simulink model "cartpole_with_obsever"  (R2023a)
settings: Solver=ode45  StartTime=0.0  StopTime=10  RelTol=1e-3
settings Model: Creator=HW  LastModifiedBy=HW

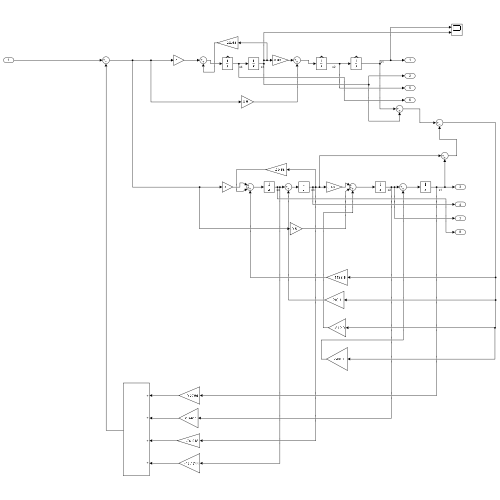
[thumbnail: Simulink's stored preview of the top-level diagram]
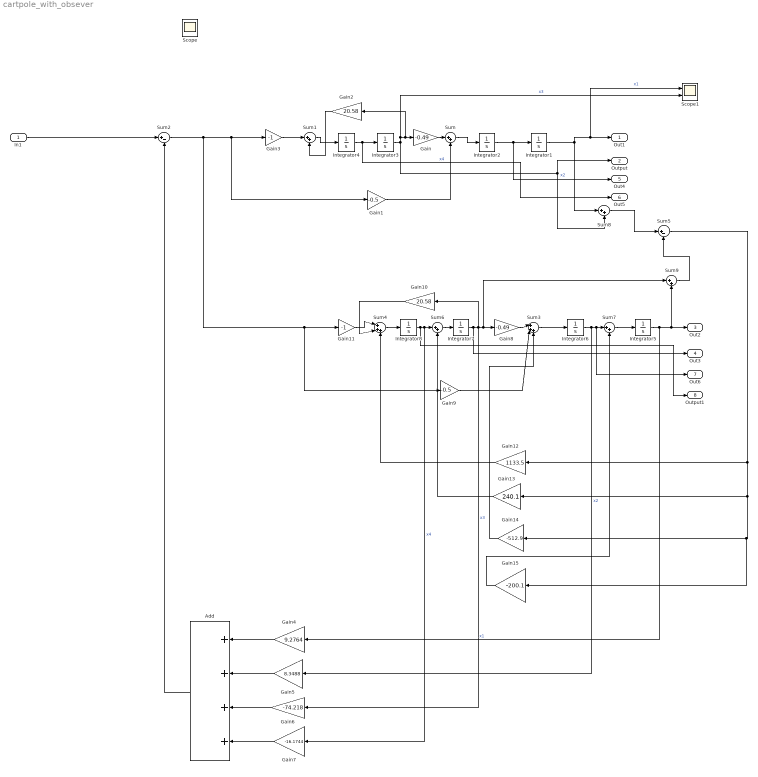
== system cartpole_with_obsever ==
  In1 : Inport
  Add : Sum  Inputs=++++
  Gain : Gain  Gain=-0.49
  Gain1 : Gain  Gain=-0.5
  Gain10 : Gain  Gain=20.58
  Gain11 : Gain  Gain=-1
  Gain12 : Gain  Gain=1133.5
  Gain13 : Gain  Gain=240.1
  Gain14 : Gain  Gain=-512.9
  Gain15 : Gain  Gain=-200.1
  Gain2 : Gain  Gain=20.58
  Gain3 : Gain  Gain=-1
  Gain4 : Gain  Gain=9.2764
  Gain5 : Gain  Gain=8.3488
  Gain6 : Gain  Gain=-74.218
  Gain7 : Gain  Gain=-16.1744
  Gain8 : Gain  Gain=-0.49
  Gain9 : Gain  Gain=-0.5
  Integrator1 : Integrator  InitialCondition=0.5  ShowStatePort=on
  Integrator2 : Integrator  InitialCondition=0.1  ShowStatePort=on
  Integrator3 : Integrator  InitialCondition=0.1
  Integrator4 : Integrator  ShowStatePort=on
  Integrator{5..8} (4 alike) : Integrator
  Scope1 : Scope  NumInputPorts=2
  Sum{,1,6..9} (6 alike) : Sum  Inputs=|++
  Sum2 : Sum  Inputs=|+-
  Sum3 : Sum  Inputs=|+++
  Sum4 : Sum  Inputs=|+++
  Sum5 : Sum  Inputs=|+-
  Out1 : Outport
  Output : Outport  Port=2
  Out2 : Outport  Port=3
  Out3 : Outport  Port=4
  Out4 : Outport  Port=5
  Out5 : Outport  Port=6
  Out6 : Outport  Port=7
  Output1 : Outport  Port=8
  Scope : Scope
  wires:
  Integrator4/1 -> Out5/1, Integrator3/1  "x4"
  Integrator2/1 -> Out4/1, Integrator1/1  "x2"
  Integrator1/1 -> Scope1/1, Out1/1, Sum8/1  "x1"
  Integrator3/1 -> Sum8/2, Output/1, Scope1/2, Gain2/1, Gain/1  "x3"
  Gain/1 -> Sum/1
  Sum/1 -> Integrator2/1
  Gain1/1 -> Sum/2
  Gain2/1 -> Sum1/2
  Sum1/1 -> Integrator4/1
  Gain3/1 -> Sum1/1
  Gain4/1 -> Add/1
  Gain5/1 -> Add/2
  Gain6/1 -> Add/3
  Gain7/1 -> Add/4
  Add/1 -> Sum2/2
  Sum2/1 -> Gain9/1, Gain11/1, Gain1/1, Gain3/1
  Sum3/1 -> Integrator6/1
  Gain10/1 -> Sum4/2
  Sum4/1 -> Integrator8/1
  Integrator5/1 -> Gain4/1, Sum9/2, Out2/1  "x1"
  Integrator8/1 -> Output1/1, Gain7/1, Sum6/1  "x4"
  Gain9/1 -> Sum3/2
  Integrator7/1 -> Out3/1, Sum9/1, Gain8/1, Gain6/1, Gain10/1  "x3"
  Gain11/1 -> Sum4/1
  Gain8/1 -> Sum3/1
  Sum5/1 -> Gain15/1, Gain14/1, Gain13/1, Gain12/1
  Gain12/1 -> Sum4/3
  Gain13/1 -> Sum6/2
  Sum6/1 -> Integrator7/1
  Gain14/1 -> Sum3/3
  Integrator6/1 -> Gain5/1, Out6/1, Sum7/1  "x2"
  Sum7/1 -> Integrator5/1
  Gain15/1 -> Sum7/2
  Sum8/1 -> Sum5/1
  Sum9/1 -> Sum5/2
  In1/1 -> Sum2/1
